simulink model "EDR100_Model3"  (R2023a)
settings: Solver=FixedStepAuto  StartTime=0  StopTime=t_end  FixedStep=h  RelTol=1e-3
InitFcn:
  | init_Model3
values from neighbouring files (symbols this model uses):
  A_f = 2.3    [Copy_of_init_Model3.m]    (also in init_Model3_allGR.m)
  c_d = 0.28    [Copy_of_init_Model3.m]    (also in init_Model3_allGR.m)
  c_r = 9.0/1000    (= 0.009)    [Copy_of_init_Model3.m]    (also in init_Model3_allGR.m)
  d_wheel = 2.101/pi*0.97    (= 0.648705998746)    [Copy_of_init_Model3.m]    (also in init_Model3_allGR.m)
  EM_inertia = 0    [Copy_of_init_Model3.m]    (also in init_Model3_allGR.m)
  EM_scaling = 1    [Copy_of_init_Model3.m]    (also in init_Model3_allGR.m)
  eta_gear = 0.98    [Copy_of_init_Model3.m]    (also in init_Model3_allGR.m)
  g = 9.81    [Copy_of_init_Model3.m]    (also in init_Model3_allGR.m)
  gear_ratio = 8    [Copy_of_init_Model3.m]    (also in init_Model3_allGR.m = 3.6:0.1:9.3; plots_model3.m = 3.6:0.1:9.3)
  h = 1.0    (= 1)    [Copy_of_init_Model3.m]    (also in import_MotorCAD_data_VL.m = surf(w,T,P_out / 1000); init_Model3_allGR.m)
  m_v = 1700    [Copy_of_init_Model3.m]    (also in init_Model3_allGR.m)
  P_aux_EM = 0    [Copy_of_init_Model3.m]    (also in init_Model3_allGR.m)
  P_aux_gear = 0    [Copy_of_init_Model3.m]    (also in init_Model3_allGR.m)
  r_wheel = d_wheel/2    (= 0.324352999373)    [Copy_of_init_Model3.m]    (also in init_Model3_allGR.m)
  rho = 1.225    [Copy_of_init_Model3.m]    (also in init_Model3_allGR.m)
  rotating_mass = 0    [Copy_of_init_Model3.m]    (also in init_Model3_allGR.m)
  T_EM = linspace(y0,y1,ny)    [Copy_of_init_Model3.m]    (also in init_Model3_allGR.m)
  T_EM_max = T_EM_raw(:,1)    [Copy_of_init_Model3.m]    (also in init_Model3_allGR.m)
  w_EM = linspace(x0,x1,nx)'    [Copy_of_init_Model3.m]    (also in init_Model3_allGR.m)
  w_EM_max = w_EM_raw(:,end)    [Copy_of_init_Model3.m]    (also in init_Model3_allGR.m)
  w_EM_upper = max(max(w_EM_raw))    [Copy_of_init_Model3.m]    (also in init_Model3_allGR.m)
settings Model: Creator=Stefan  LastModifiedBy=victo
settings OptimizationCC: ReuseModelBlockBuffer=off
settings DebuggingCC: UnconnectedInputMsg=warning  UnconnectedOutputMsg=warning  UnconnectedLineMsg=warning
settings ModelReferenceCC: EnableRefExpFcnMdlSchedulingChecks=on
settings RTWCC: DLArmComputeVersion=19.05

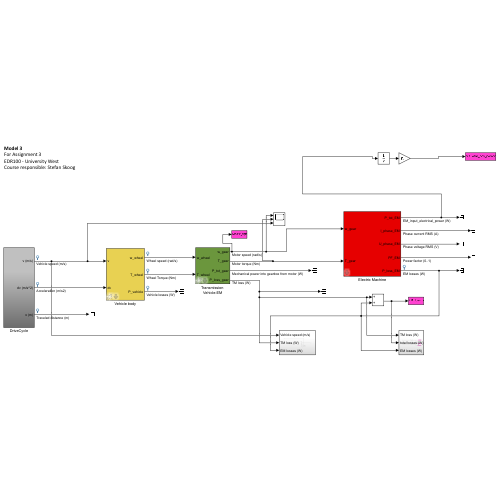
[thumbnail: Simulink's stored preview of the top-level diagram]
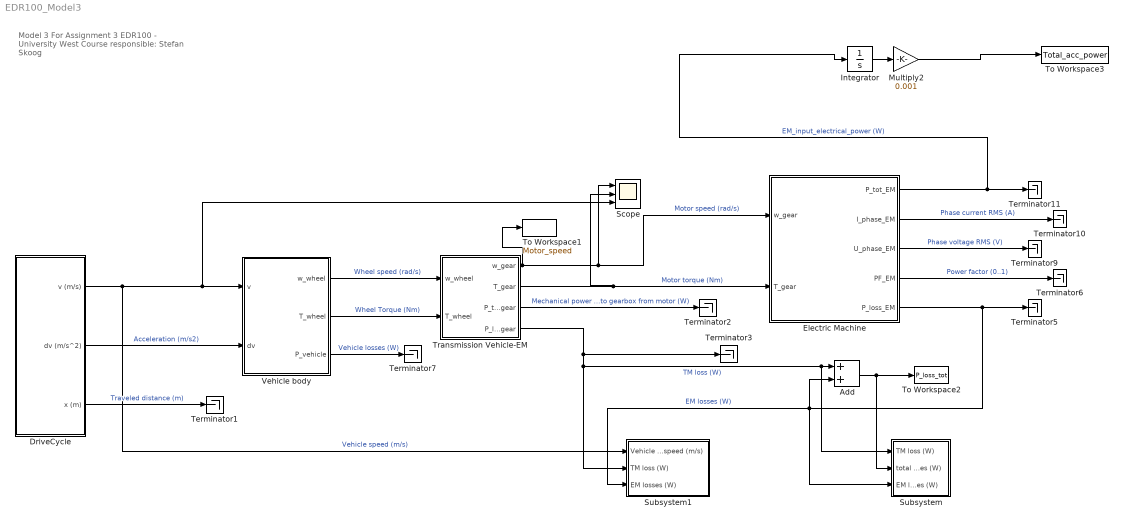
== system EDR100_Model3 ==
  note: Model 3
      | For Assignment 3
      | EDR100 - University West
      | Course responsible: Stefan Skoog
  Add : Sum
  DriveCycle : Subsystem
  Electric Machine : Subsystem  mask{scale_EM=EM_scaling, theta_EM=EM_inertia, EM_P_aux=P_aux_EM}
      mask prompts: scale_EM "EM Scaling Factor (-)"; theta_EM "EM Inertia (kg*m²)"; EM_P_aux "Aux power (W)"
  Integrator : Integrator
  Multiply2 : Gain  Gain=0.001
  Scope : Scope  NumInputPorts=3
  Subsystem : Subsystem
  Subsystem1 : Subsystem
  Terminator{1..3,5..7,9..11} (9 alike) : Terminator
  To Workspace1 : ToWorkspace  VariableName=Motor_speed  SampleTime=-1
      settings: Save2DSignal=2-D array (concatenate along first dimension)
  To Workspace2 : ToWorkspace  VariableName=P_loss_tot  SampleTime=-1
      settings: Save2DSignal=2-D array (concatenate along first dimension)
  To Workspace3 : ToWorkspace  VariableName=Total_acc_power  SampleTime=-1
      settings: Save2DSignal=2-D array (concatenate along first dimension)
  Transmission Vehicle-EM : Subsystem  Tag=simple transmission  AncestorBlock=qss_tb_library/Gear System/Transmission  mask(Transmission){gear_ratio=gear_ratio, e_GT=eta_gear, P_GT0=P_aux_gear, w_wheel_min=1}
      mask prompts: gear_ratio "Gear ratio [-]"; e_GT "Efficiency [-]"; P_GT0 "Idling losses (friction) [W]"; w_wheel_min "Minimum wheel speed beyond which losses are generated [rad/s]"
      mask help:
      | This block simulates a transmission with a fixed gear ratio.
      |
      | Input:
      | =====
      | 	w_wheel	Speed of the wheel [rad/s]
      | 	dw_wheel	Acceleration of the wheel [rad/s^2]
      | 	T_wheel	Torque on the wheel [Nm]
      |
      | Output:
      | ======
      | 	w_trans		Speed of the fly wheel [rad/s]
      | 	dw_trans	Acceleration of the fly wheel [rad/s^2]
      | 	T_trans		Torque on the fly wheel [Nm]
  Vehicle body : Subsystem  Tag=vehicle  AncestorBlock=qss_tb_library/Vehicle/Vehicle  mask(Vehicle){m_f=m_v, mt2m_f=rotating_mass, A_f=A_f, d_wheel=d_wheel, cw=c_d, mu=c_r}
      mask prompts: m_f "Total mass of the vehicle [kg]"; mt2m_f "Rotating mass [%]"; A_f "Vehicle cross section [m^2]"; d_wheel "Wheel diameter [m]"; cw "Drag coefficient [-]"; mu "Rolling friction coefficient [-]"
      mask help:
      | This block computes the power required from the vehicle.
      |
      | Input:
      | =====
      | 	v		Speed [m/s]
      | 	dv		Acceleration [m/s^2]
      |
      | Output:
      | ======
      | 	w_wheel	Speed of the wheel [rad/s]
      | 	dw_wheel	Acceleration of the wheel [rad/s^2]
      | 	T_wheel	Torque on the wheel [Nm]
  wires:
  DriveCycle/2(dv (m/s^2)) -> Vehicle body/2(dv)  "Acceleration (m/s2)"
  DriveCycle/1(v (m/s)) -> Subsystem1/1(Vehicle speed (m/s)), Scope/3, Vehicle body/1(v)  "Vehicle speed (m/s)"
  Vehicle body/1(w_wheel) -> Transmission Vehicle-EM/1(w_wheel)  "Wheel speed (rad/s)"
  Vehicle body/2(T_wheel) -> Transmission Vehicle-EM/2(T_wheel)  "Wheel Torque (Nm)"
  Vehicle body/3(P_vehicle) -> Terminator7/1  "Vehicle losses (W)"
  DriveCycle/3(x (m)) -> Terminator1/1  "Traveled distance (m)"
  Transmission Vehicle-EM/3(P_tot_gear) -> Terminator2/1  "Mechanical power into gearbox from motor (W)"
  Transmission Vehicle-EM/4(P_loss_gear) -> Subsystem1/2(TM loss (W)), Subsystem/1(TM loss (W)), Add/1, Terminator3/1  "TM loss (W)"
  Transmission Vehicle-EM/2(T_gear) -> Scope/2, Electric Machine/2(T_gear)  "Motor torque (Nm)"
  Transmission Vehicle-EM/1(w_gear) -> To Workspace1/1, Scope/1, Electric Machine/1(w_gear)  "Motor speed (rad/s)"
  Electric Machine/5(P_loss_EM) -> Subsystem1/3(EM losses (W)), Subsystem/3(EM losses (W)), Add/2, Terminator5/1  "EM losses (W)"
  Electric Machine/4(PF_EM) -> Terminator6/1  "Power factor (0..1)"
  Electric Machine/3(U_phase_EM) -> Terminator9/1  "Phase voltage RMS (V)"
  Electric Machine/2(I_phase_EM) -> Terminator10/1  "Phase current RMS (A)"
  Electric Machine/1(P_tot_EM) -> Integrator/1, Terminator11/1  "EM_input_electrical_power (W)"
  Add/1 -> Subsystem/2(total losses (W)), To Workspace2/1
  Multiply2/1 -> To Workspace3/1
  Integrator/1 -> Multiply2/1

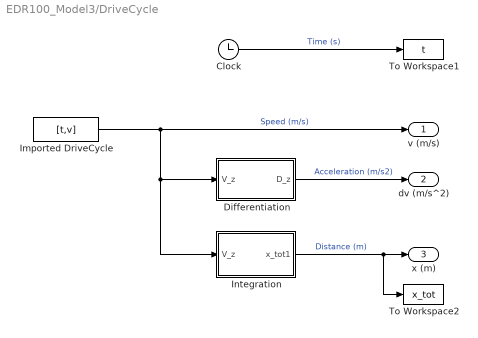
== system EDR100_Model3/DriveCycle ==
  Clock : Clock
  Differentiation : Subsystem
  Imported DriveCycle : FromWorkspace  VariableName=[t,v]  SampleTime=h  OutputAfterFinalValue=Setting to zero
  Integration : Subsystem
  To Workspace1 : ToWorkspace  VariableName=t  SampleTime=-1
  To Workspace2 : ToWorkspace  VariableName=x_tot  SampleTime=-1
  v (m/s) : Outport
  dv (m/s^2) : Outport  Port=2
  x (m) : Outport  Port=3  InitialOutput=0
  wires:
  Clock/1 -> To Workspace1/1  "Time (s)"
  Imported DriveCycle/1 -> Differentiation/1(V_z), Integration/1(V_z), v (m/s)/1  "Speed (m/s)"
  Integration/1(x_tot1) -> To Workspace2/1, x (m)/1  "Distance (m)"
  Differentiation/1(D_z) -> dv (m/s^2)/1  "Acceleration (m/s2)"

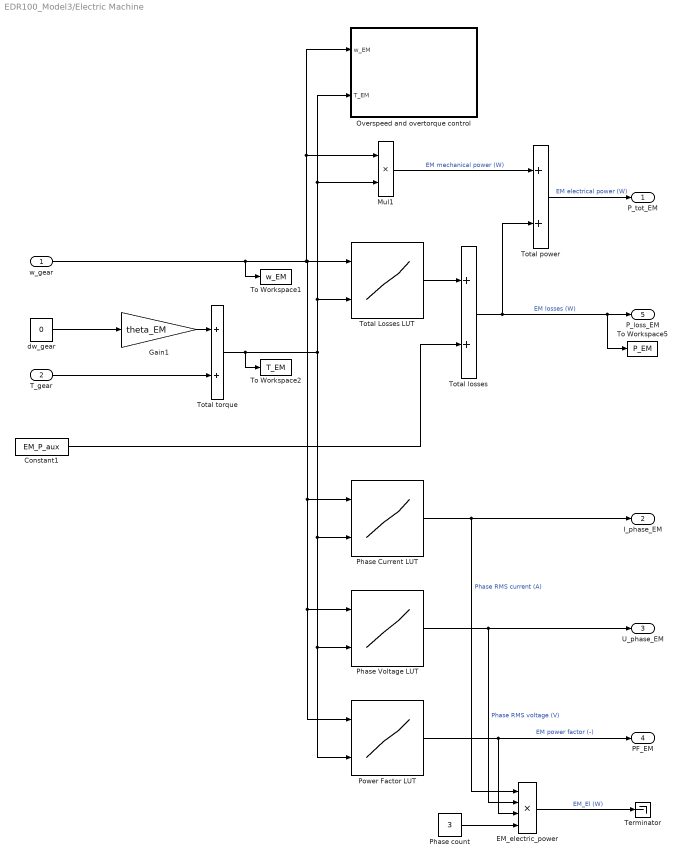
== system EDR100_Model3/Electric Machine ==
  w_gear : Inport
  T_gear : Inport  Port=2
  Constant1 : Constant  Value=EM_P_aux
  EM_electric_power : Product  Inputs=4
  Gain1 : Gain  Gain=theta_EM  SaturateOnIntegerOverflow=on  OutDataTypeStr=Inherit: Same as input  ParamDataTypeStr=Inherit: Same as input
  Mul1 : Product  Inputs=**
  Overspeed and overtorque control : Subsystem
  Phase Current LUT : Lookup_n-D  BreakpointsForDimension1=w_EM  BreakpointsForDimension2=T_EM  Table=Iph_EM_map'  ExtrapMethod=Clip  InternalRulePriority=Speed  RndMeth=Simplest
      settings: InputPortMap=u0,u1
  Phase Voltage LUT : Lookup_n-D  BreakpointsForDimension1=w_EM  BreakpointsForDimension2=T_EM  Table=Uph_EM_map'  ExtrapMethod=Clip  InternalRulePriority=Speed  RndMeth=Simplest
      settings: InputPortMap=u0,u1
  Phase count : Constant  Value=3
  Power Factor LUT : Lookup_n-D  BreakpointsForDimension1=w_EM  BreakpointsForDimension2=T_EM  Table=PF_EM_map'  ExtrapMethod=Clip  InternalRulePriority=Speed  RndMeth=Simplest
      settings: InputPortMap=u0,u1
  Terminator : Terminator
  To Workspace1 : ToWorkspace  VariableName=w_EM  SampleTime=-1
  To Workspace2 : ToWorkspace  VariableName=T_EM  SampleTime=-1
  To Workspace5 : ToWorkspace  VariableName=P_EM  SampleTime=-1
  Total Losses LUT : Lookup_n-D  BreakpointsForDimension1=w_EM  BreakpointsForDimension2=T_EM  Table=Loss_EM_map'  ExtrapMethod=Clip  InternalRulePriority=Speed  RndMeth=Simplest
      settings: InputPortMap=u0,u1
  Total losses : Sum  InputSameDT=on  SaturateOnIntegerOverflow=on  OutDataTypeStr=Inherit: Same as first input
  Total power : Sum  InputSameDT=on  SaturateOnIntegerOverflow=on  OutDataTypeStr=Inherit: Same as first input
  Total torque : Sum  InputSameDT=on  SaturateOnIntegerOverflow=on  OutDataTypeStr=Inherit: Same as first input
  dw_gear : Constant  Value=0
  P_tot_EM : Outport
  I_phase_EM : Outport  Port=2
  U_phase_EM : Outport  Port=3
  PF_EM : Outport  Port=4
  P_loss_EM : Outport  Port=5
  wires:
  T_gear/1 -> Total torque/2
  dw_gear/1 -> Gain1/1
  w_gear/1 -> To Workspace1/1, Total Losses LUT/1, Phase Current LUT/1, Power Factor LUT/1, Phase Voltage LUT/1, Overspeed and overtorque control/1(w_EM), Mul1/1
  Total losses/1 -> Total power/2, P_loss_EM/1, To Workspace5/1  "EM losses (W)"
  Total Losses LUT/1 -> Total losses/1
  Gain1/1 -> Total torque/1
  Total torque/1 -> Phase Current LUT/2, Power Factor LUT/2, Phase Voltage LUT/2, Total Losses LUT/2, Overspeed and overtorque control/2(T_EM), Mul1/2, To Workspace2/1
  Constant1/1 -> Total losses/2
  Phase Current LUT/1 -> I_phase_EM/1, EM_electric_power/1  "Phase RMS current (A)"
  Phase Voltage LUT/1 -> U_phase_EM/1, EM_electric_power/2  "Phase RMS voltage (V)"
  Total power/1 -> P_tot_EM/1  "EM electrical power (W)"
  Mul1/1 -> Total power/1  "EM mechanical power (W)"
  Power Factor LUT/1 -> PF_EM/1, EM_electric_power/3  "EM power factor (-)"
  EM_electric_power/1 -> Terminator/1  "EM_El (W)"
  Phase count/1 -> EM_electric_power/4

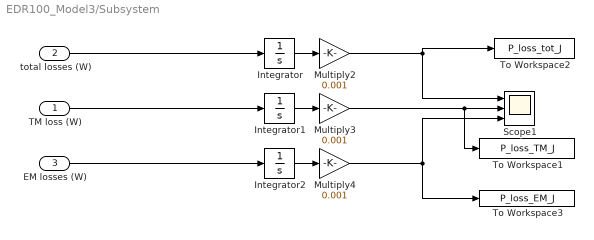
== system EDR100_Model3/Subsystem ==
  TM loss (W) : Inport
  total losses (W) : Inport  Port=2
  EM losses (W) : Inport  Port=3
  Integrator : Integrator
  Integrator1 : Integrator
  Integrator2 : Integrator
  Multiply2 : Gain  Gain=0.001
  Multiply3 : Gain  Gain=0.001
  Multiply4 : Gain  Gain=0.001
  Scope1 : Scope  NumInputPorts=3
  To Workspace1 : ToWorkspace  VariableName=P_loss_TM_J  SampleTime=-1
      settings: Save2DSignal=2-D array (concatenate along first dimension)
  To Workspace2 : ToWorkspace  VariableName=P_loss_tot_J  SampleTime=-1
      settings: Save2DSignal=2-D array (concatenate along first dimension)
  To Workspace3 : ToWorkspace  VariableName=P_loss_EM_J  SampleTime=-1
      settings: Save2DSignal=2-D array (concatenate along first dimension)
  wires:
  total losses (W)/1 -> Integrator/1
  TM loss (W)/1 -> Integrator1/1
  Integrator2/1 -> Multiply4/1
  Integrator1/1 -> Multiply3/1
  Integrator/1 -> Multiply2/1
  Multiply2/1 -> To Workspace2/1, Scope1/1
  Multiply3/1 -> To Workspace1/1, Scope1/2
  Multiply4/1 -> To Workspace3/1, Scope1/3
  EM losses (W)/1 -> Integrator2/1

== system EDR100_Model3/Subsystem1 ==
  Vehicle speed (m/s) : Inport
  TM loss (W) : Inport  Port=2
  EM losses (W) : Inport  Port=3
  Multiply : Gain  Gain=0.001
  Multiply1 : Gain  Gain=0.001
  Scope : Scope  NumInputPorts=3
  wires:
  Multiply/1 -> Scope/2
  Multiply1/1 -> Scope/3
  Vehicle speed (m/s)/1 -> Scope/1
  EM losses (W)/1 -> Multiply1/1
  TM loss (W)/1 -> Multiply/1

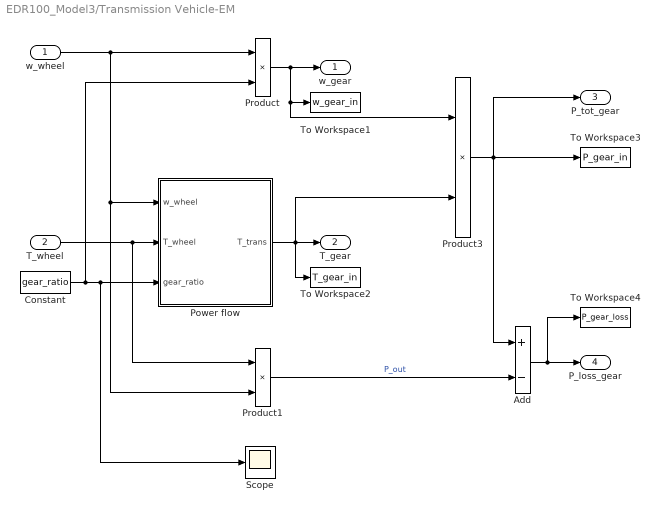
== system EDR100_Model3/Transmission Vehicle-EM ==
  w_wheel : Inport
  T_wheel : Inport  Port=2
  Add : Sum  Inputs=+-
  Constant : Constant  Value=gear_ratio
  Power flow : Subsystem
  Product : Product  InputSameDT=on  RndMeth=Zero  SaturateOnIntegerOverflow=on  OutDataTypeStr=Inherit: Same as first input
  Product1 : Product  InputSameDT=on  RndMeth=Zero  SaturateOnIntegerOverflow=on  OutDataTypeStr=Inherit: Same as first input
  Product3 : Product  InputSameDT=on  RndMeth=Zero  SaturateOnIntegerOverflow=on  OutDataTypeStr=Inherit: Same as first input
  Scope : Scope
  To Workspace1 : ToWorkspace  VariableName=w_gear_in  SampleTime=-1
  To Workspace2 : ToWorkspace  VariableName=T_gear_in  SampleTime=-1
  To Workspace3 : ToWorkspace  VariableName=P_gear_in  SampleTime=-1
  To Workspace4 : ToWorkspace  VariableName=P_gear_loss  SampleTime=-1
  w_gear : Outport  InitialOutput=0
  T_gear : Outport  Port=2  InitialOutput=0
  P_tot_gear : Outport  Port=3  InitialOutput=0
  P_loss_gear : Outport  Port=4  InitialOutput=0
  wires:
  Product3/1 -> P_tot_gear/1, To Workspace3/1, Add/1
  w_wheel/1 -> Product1/2, Power flow/1(w_wheel), Product/1
  Constant/1 -> Product/2, Scope/1, Power flow/3(gear_ratio)
  T_wheel/1 -> Product1/1, Power flow/2(T_wheel)
  Product/1 -> Product3/1, To Workspace1/1, w_gear/1
  Power flow/1(T_trans) -> Product3/2, To Workspace2/1, T_gear/1
  Product1/1 -> Add/2  "P_out"
  Add/1 -> To Workspace4/1, P_loss_gear/1

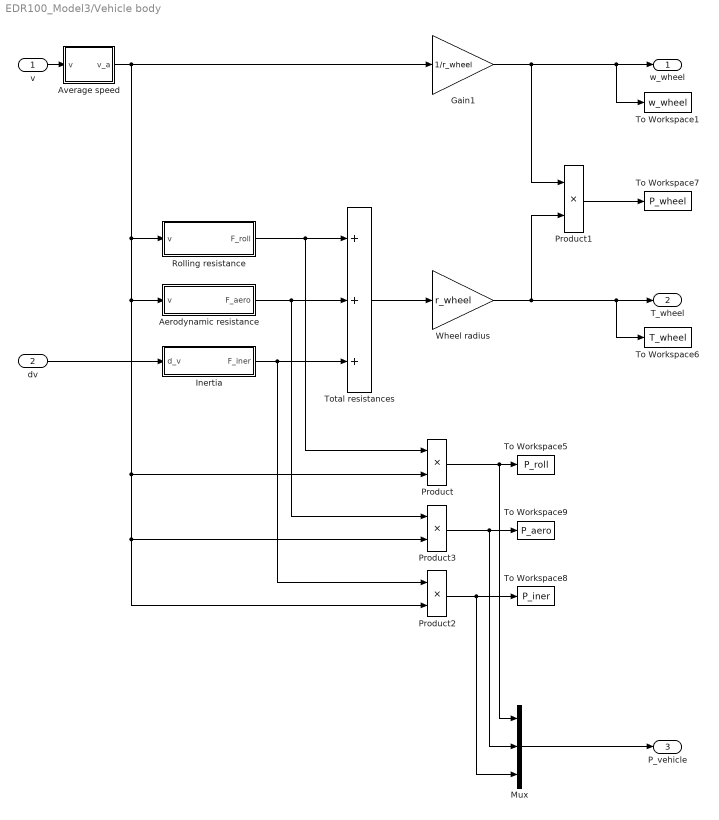
== system EDR100_Model3/Vehicle body ==
  v : Inport
  dv : Inport  Port=2
  Aerodynamic resistance : Subsystem
  Average speed : Subsystem
  Gain1 : Gain  Gain=1/r_wheel  SaturateOnIntegerOverflow=on  OutDataTypeStr=Inherit: Same as input  ParamDataTypeStr=Inherit: Same as input
  Inertia : Subsystem
  Mux : Mux  Inputs=3
  Product{,1..3} (4 alike) : Product  InputSameDT=on  RndMeth=Zero  SaturateOnIntegerOverflow=on  OutDataTypeStr=Inherit: Same as first input
  Rolling resistance : Subsystem
  To Workspace1 : ToWorkspace  VariableName=w_wheel  SampleTime=-1
  To Workspace5 : ToWorkspace  VariableName=P_roll  SampleTime=-1
  To Workspace6 : ToWorkspace  VariableName=T_wheel  SampleTime=-1
  To Workspace7 : ToWorkspace  VariableName=P_wheel  SampleTime=-1
  To Workspace8 : ToWorkspace  VariableName=P_iner  SampleTime=-1
  To Workspace9 : ToWorkspace  VariableName=P_aero  SampleTime=-1
  Total resistances : Sum  Inputs=+++  InputSameDT=on  SaturateOnIntegerOverflow=on  OutDataTypeStr=Inherit: Same as first input
  Wheel radius : Gain  Gain=r_wheel  SaturateOnIntegerOverflow=on  OutDataTypeStr=Inherit: Same as input  ParamDataTypeStr=Inherit: Same as input
  w_wheel : Outport  InitialOutput=0
  T_wheel : Outport  Port=2  InitialOutput=0
  P_vehicle : Outport  Port=3  InitialOutput=0
  wires:
  Product/1 -> Mux/1, To Workspace5/1
  Product1/1 -> To Workspace7/1
  Product3/1 -> Mux/2, To Workspace9/1
  Product2/1 -> Mux/3, To Workspace8/1
  v/1 -> Average speed/1(v)
  dv/1 -> Inertia/1(d_v)
  Wheel radius/1 -> Product1/2, To Workspace6/1, T_wheel/1
  Total resistances/1 -> Wheel radius/1
  Inertia/1(F_iner) -> Product2/1, Total resistances/3
  Aerodynamic resistance/1(F_aero) -> Total resistances/2, Product3/1
  Rolling resistance/1(F_roll) -> Product/1, Total resistances/1
  Gain1/1 -> To Workspace1/1, w_wheel/1, Product1/1
  Average speed/1(v_a) -> Product/2, Product2/2, Product3/2, Aerodynamic resistance/1(v), Rolling resistance/1(v), Gain1/1
  Mux/1 -> P_vehicle/1

== system EDR100_Model3/DriveCycle/Differentiation ==
  V_z : Inport
  Sum1 : Sum  Inputs=+-  InputSameDT=on  SaturateOnIntegerOverflow=on  OutDataTypeStr=Inherit: Same as first input
  Unit Delay1 : UnitDelay  SampleTime=h
  D_z : Outport  InitialOutput=0
  wires:
  Unit Delay1/1 -> Sum1/2
  V_z/1 -> Sum1/1, Unit Delay1/1
  Sum1/1 -> D_z/1

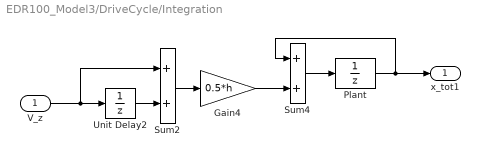
== system EDR100_Model3/DriveCycle/Integration ==
  V_z : Inport
  Gain4 : Gain  Gain=0.5*h  SaturateOnIntegerOverflow=on  OutDataTypeStr=Inherit: Same as input  ParamDataTypeStr=Inherit: Same as input
  Plant : UnitDelay  InitialCondition=1  SampleTime=h
  Sum2 : Sum  InputSameDT=on  SaturateOnIntegerOverflow=on  OutDataTypeStr=Inherit: Same as first input
  Sum4 : Sum  InputSameDT=on  SaturateOnIntegerOverflow=on  OutDataTypeStr=Inherit: Same as first input
  Unit Delay2 : UnitDelay  SampleTime=h
  x_tot1 : Outport  InitialOutput=0
  wires:
  Unit Delay2/1 -> Sum2/2
  Sum2/1 -> Gain4/1
  Gain4/1 -> Sum4/2
  Plant/1 -> x_tot1/1, Sum4/1
  V_z/1 -> Sum2/1, Unit Delay2/1
  Sum4/1 -> Plant/1

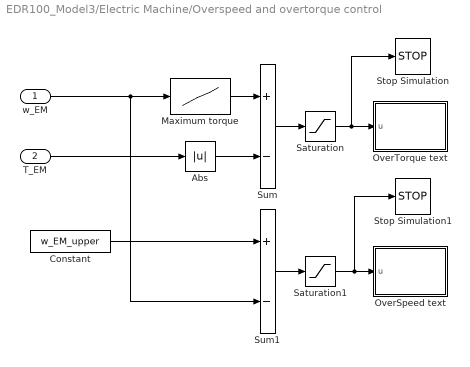
== system EDR100_Model3/Electric Machine/Overspeed and overtorque control ==
  w_EM : Inport
  T_EM : Inport  Port=2
  Abs : Abs
  Constant : Constant  Value=w_EM_upper
  Maximum torque : Lookup  InputValues=w_EM_max  Table=T_EM_max
  OverSpeed text : MATLAB Function  TreatAsAtomicUnit=on
  OverTorque text : MATLAB Function  TreatAsAtomicUnit=on
  Saturation : Saturate  UpperLimit=0  LowerLimit=-inf
  Saturation1 : Saturate  UpperLimit=0  LowerLimit=-inf
  Stop Simulation : Stop
  Stop Simulation1 : Stop
  Sum : Sum  Inputs=+-  InputSameDT=on  SaturateOnIntegerOverflow=on  OutDataTypeStr=Inherit: Same as first input
  Sum1 : Sum  Inputs=+-  InputSameDT=on  SaturateOnIntegerOverflow=on  OutDataTypeStr=Inherit: Same as first input
  wires:
  Saturation/1 -> Stop Simulation/1, OverTorque text/1(u)
  Constant/1 -> Sum1/1
  w_EM/1 -> Maximum torque/1, Sum1/2
  Abs/1 -> Sum/2
  Saturation1/1 -> Stop Simulation1/1, OverSpeed text/1(u)
  Sum1/1 -> Saturation1/1
  T_EM/1 -> Abs/1
  Maximum torque/1 -> Sum/1
  Sum/1 -> Saturation/1

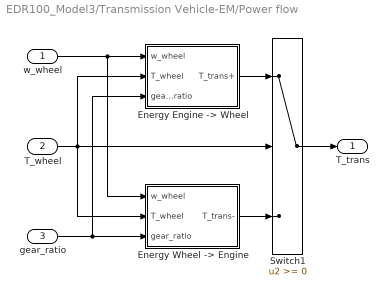
== system EDR100_Model3/Transmission Vehicle-EM/Power flow ==
  w_wheel : Inport
  T_wheel : Inport  Port=2
  gear_ratio : Inport  Port=3
  "Energy Engine -> Wheel" : Subsystem
  "Energy Wheel -> Engine" : Subsystem
  Switch1 : Switch
  T_trans : Outport  InitialOutput=0
  wires:
  Switch1/1 -> T_trans/1
  "Energy Engine -> Wheel"/1(T_trans+) -> Switch1/1
  T_wheel/1 -> Switch1/2, "Energy Engine -> Wheel"/2(T_wheel), "Energy Wheel -> Engine"/2(T_wheel)
  "Energy Wheel -> Engine"/1(T_trans-) -> Switch1/3
  gear_ratio/1 -> "Energy Engine -> Wheel"/3(gear_ratio), "Energy Wheel -> Engine"/3(gear_ratio)
  w_wheel/1 -> "Energy Engine -> Wheel"/1(w_wheel), "Energy Wheel -> Engine"/1(w_wheel)

== system EDR100_Model3/Vehicle body/Aerodynamic resistance ==
  v : Inport
  Aerodynamic resistance : Fcn  Expr=0.5*rho*cw*A_f*u^2
  To Workspace10 : ToWorkspace  VariableName=F_aero  SampleTime=-1
  F_aero : Outport  InitialOutput=0
  wires:
  Aerodynamic resistance/1 -> To Workspace10/1, F_aero/1
  v/1 -> Aerodynamic resistance/1

== system EDR100_Model3/Vehicle body/Average speed ==
  v : Inport
  Gain5 : Gain  Gain=0.5  SaturateOnIntegerOverflow=on  OutDataTypeStr=Inherit: Same as input  ParamDataTypeStr=Inherit: Same as input
  Sum2 : Sum  InputSameDT=on  SaturateOnIntegerOverflow=on  OutDataTypeStr=Inherit: Same as first input
  Unit Delay : UnitDelay  SampleTime=h
  v_a : Outport  InitialOutput=0
  wires:
  v/1 -> Unit Delay/1, Sum2/1
  Gain5/1 -> v_a/1
  Sum2/1 -> Gain5/1
  Unit Delay/1 -> Sum2/2

== system EDR100_Model3/Vehicle body/Inertia ==
  d_v : Inport
  Inertia : Fcn  Expr=m_f*(1+mt2m_f)*u/h
  To Workspace10 : ToWorkspace  VariableName=F_iner  SampleTime=-1
  F_iner : Outport  InitialOutput=0
  wires:
  d_v/1 -> Inertia/1
  Inertia/1 -> To Workspace10/1, F_iner/1

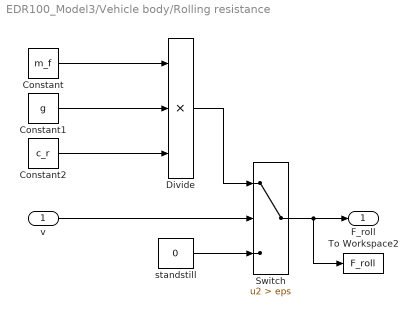
== system EDR100_Model3/Vehicle body/Rolling resistance ==
  v : Inport
  Constant : Constant  Value=m_f
  Constant1 : Constant  Value=g
  Constant2 : Constant  Value=c_r
  Divide : Product  Inputs=***
  Switch : Switch  Criteria=u2 > Threshold  Threshold=eps  SaturateOnIntegerOverflow=off  InputSameDT=off
  To Workspace2 : ToWorkspace  VariableName=F_roll  SampleTime=-1
  standstill : Constant  Value=0
  F_roll : Outport
  wires:
  standstill/1 -> Switch/3
  v/1 -> Switch/2
  Switch/1 -> F_roll/1, To Workspace2/1
  Constant/1 -> Divide/1
  Constant1/1 -> Divide/2
  Constant2/1 -> Divide/3
  Divide/1 -> Switch/1

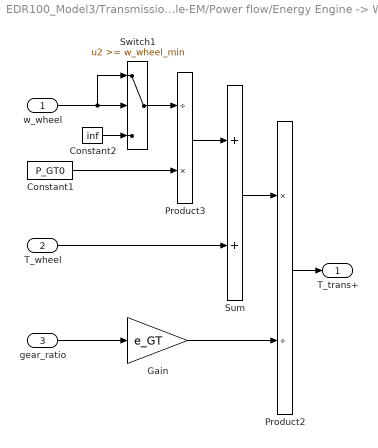
== system EDR100_Model3/Transmission Vehicle-EM/Power flow/Energy Engine -> Wheel ==
  w_wheel : Inport
  T_wheel : Inport  Port=2
  gear_ratio : Inport  Port=3
  Constant1 : Constant  Value=P_GT0
  Constant2 : Constant  Value=inf
  Gain : Gain  Gain=e_GT  SaturateOnIntegerOverflow=on  OutDataTypeStr=Inherit: Same as input  ParamDataTypeStr=Inherit: Same as input
  Product2 : Product  Inputs=*/  InputSameDT=on  RndMeth=Zero  SaturateOnIntegerOverflow=on  OutDataTypeStr=Inherit: Same as first input
  Product3 : Product  Inputs=/*  InputSameDT=on  RndMeth=Zero  SaturateOnIntegerOverflow=on  OutDataTypeStr=Inherit: Same as first input
  Sum : Sum  InputSameDT=on  SaturateOnIntegerOverflow=on  OutDataTypeStr=Inherit: Same as first input
  Switch1 : Switch  Threshold=w_wheel_min
  T_trans+ : Outport  InitialOutput=0
  wires:
  gear_ratio/1 -> Gain/1
  Constant1/1 -> Product3/2
  Switch1/1 -> Product3/1
  Constant2/1 -> Switch1/3
  w_wheel/1 -> Switch1/1, Switch1/2
  Sum/1 -> Product2/1
  Product2/1 -> T_trans+/1
  Gain/1 -> Product2/2
  Product3/1 -> Sum/1
  T_wheel/1 -> Sum/2

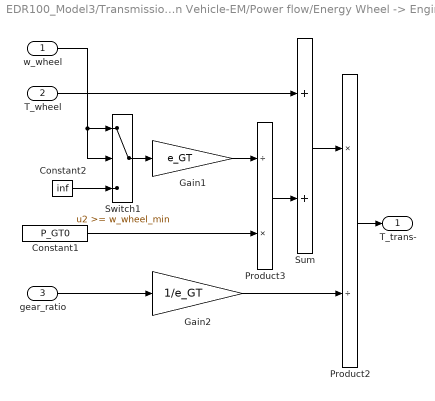
== system EDR100_Model3/Transmission Vehicle-EM/Power flow/Energy Wheel -> Engine ==
  w_wheel : Inport
  T_wheel : Inport  Port=2
  gear_ratio : Inport  Port=3
  Constant1 : Constant  Value=P_GT0
  Constant2 : Constant  Value=inf
  Gain1 : Gain  Gain=e_GT  SaturateOnIntegerOverflow=on  OutDataTypeStr=Inherit: Same as input  ParamDataTypeStr=Inherit: Same as input
  Gain2 : Gain  Gain=1/e_GT  SaturateOnIntegerOverflow=on  OutDataTypeStr=Inherit: Same as input  ParamDataTypeStr=Inherit: Same as input
  Product2 : Product  Inputs=*/  InputSameDT=on  RndMeth=Zero  SaturateOnIntegerOverflow=on  OutDataTypeStr=Inherit: Same as first input
  Product3 : Product  Inputs=/*  InputSameDT=on  RndMeth=Zero  SaturateOnIntegerOverflow=on  OutDataTypeStr=Inherit: Same as first input
  Sum : Sum  InputSameDT=on  SaturateOnIntegerOverflow=on  OutDataTypeStr=Inherit: Same as first input
  Switch1 : Switch  Threshold=w_wheel_min
  T_trans- : Outport  InitialOutput=0
  wires:
  Gain1/1 -> Product3/1
  Sum/1 -> Product2/1
  Product3/1 -> Sum/2
  Product2/1 -> T_trans-/1
  Gain2/1 -> Product2/2
  T_wheel/1 -> Sum/1
  Constant1/1 -> Product3/2
  Switch1/1 -> Gain1/1
  Constant2/1 -> Switch1/3
  gear_ratio/1 -> Gain2/1
  w_wheel/1 -> Switch1/2, Switch1/1

== matlab function EDR100_Model3/Electric Machine/Overspeed and overtorque control/OverTorque text ==
  data: u input
function fcn(u)
    if u ~ 0
        %error('EM over-torque error! \n');
        fprintf(2, 'EM over-torque error! \n');
    end
end

== matlab function EDR100_Model3/Electric Machine/Overspeed and overtorque control/OverSpeed text ==
  data: u input
    function fcn(u)
    if u ~ 0
        %error('EM over-speed error!');
        fprintf(2, 'EM over-speed error! \n');
    end
end
